simulink model "fuzzy_controller"  (R2015a)
settings: Solver=ode45  StartTime=0.0  StopTime=5  RelTol=1e-3
PreLoadFcn:
  | fuzzy_logic
InitFcn:
  | fuzzy_logic
StartFcn:
  | fuzzy_logic
values from neighbouring files (symbols this model uses):
  A = [zeros(3,3) eye(3); -inv(D_)*G zeros(3,3)]    [double_pend_feedback.m]    (also in fuzzy_logic.m = [zeros(3,3) eye(3); inv(D_)*G zeros(3,3)]; single_pend.m = [0 1 0 0; (g*(M+m))/(l*M) 0 0 b/(l*M); 0 0 0 1; -m*g/M 0 0 -)
  B = [zeros(3,1); inv(D_)*H]    [double_pend_feedback.m]    (also in fuzzy_logic.m; single_pend.m = [0;-1/(l*M); 0 ; 1/M])
  K = double([sol.k1,sol.k2,sol.k3,sol.k4,sol.k5,sol.k6])    [double_pend_feedback.m]    (also in fuzzy_logic.m = lqr2; single_pend.m = [k1 k2 k3 k4])
libraries: fuzblock x1
settings Model: Creator=Nabeel  LastModifiedBy=Nabeel

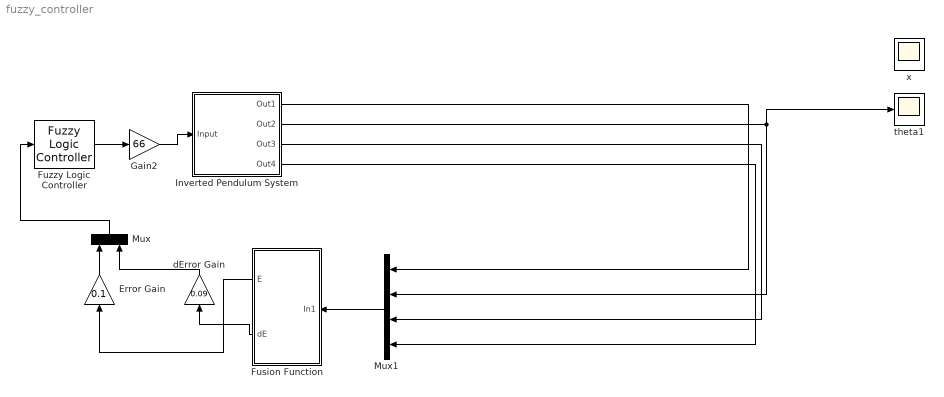
== system fuzzy_controller ==
  Error Gain : Gain  Gain=0.1
  Fusion Function : Subsystem
  Fuzzy Logic Controller : fuzblock/Fuzzy Logic  Controller  fis='MYFUZ.fis'
  Gain2 : Gain  Gain=66
  Inverted Pendulum System : Subsystem
  Mux : Mux  Inputs=2
  Mux1 : Mux
  dError Gain : Gain  Gain=0.09
  theta1 : Scope
      settings: SaveName=theta1
  x : Scope
      settings: SaveName=x
  wires:
  Fuzzy Logic Controller/1 -> Gain2/1
  Gain2/1 -> Inverted Pendulum System/1(Input)
  Fusion Function/1(E) -> Error Gain/1
  Fusion Function/2(dE) -> dError Gain/1
  Mux/1 -> Fuzzy Logic Controller/1
  Error Gain/1 -> Mux/1
  dError Gain/1 -> Mux/2
  Mux1/1 -> Fusion Function/1(In1)
  Inverted Pendulum System/1(Out1) -> Mux1/1
  Inverted Pendulum System/2(Out2) -> Mux1/2, theta1/1
  Inverted Pendulum System/3(Out3) -> Mux1/3
  Inverted Pendulum System/4(Out4) -> Mux1/4

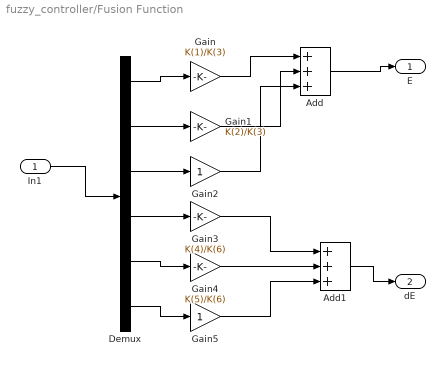
== system fuzzy_controller/Fusion Function ==
  In1 : Inport
  Add : Sum  Inputs=+++
  Add1 : Sum  Inputs=+++
  Demux : Demux  Outputs=6
  Gain : Gain  Gain=K(1)/K(3)
  Gain1 : Gain  Gain=K(2)/K(3)
  Gain2 : Gain
  Gain3 : Gain  Gain=K(4)/K(6)
  Gain4 : Gain  Gain=K(5)/K(6)
  Gain5 : Gain
  E : Outport
  dE : Outport  Port=2
  wires:
  In1/1 -> Demux/1
  Add1/1 -> dE/1
  Add/1 -> E/1
  Demux/6 -> Gain5/1
  Demux/5 -> Gain4/1
  Demux/4 -> Gain3/1
  Demux/3 -> Gain2/1
  Demux/2 -> Gain1/1
  Demux/1 -> Gain/1
  Gain3/1 -> Add1/1
  Gain4/1 -> Add1/2
  Gain5/1 -> Add1/3
  Gain2/1 -> Add/3
  Gain1/1 -> Add/2
  Gain/1 -> Add/1

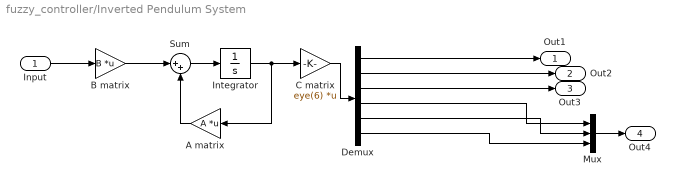
== system fuzzy_controller/Inverted Pendulum System ==
  Input : Inport
  A matrix : Gain  Gain=A  Multiplication=Matrix(K*u)
  B matrix : Gain  Gain=B  Multiplication=Matrix(K*u)
  C matrix : Gain  Gain=eye(6)  Multiplication=Matrix(K*u)
  Demux : Demux  Outputs=6
  Integrator : Integrator  InitialCondition=[0 0.1 0.1 0 0 0]
  Mux : Mux  Inputs=3
  Sum : Sum  Inputs=|++
  Out1 : Outport
  Out2 : Outport  Port=2
  Out3 : Outport  Port=3
  Out4 : Outport  Port=4
  wires:
  Input/1 -> B matrix/1
  A matrix/1 -> Sum/2
  B matrix/1 -> Sum/1
  Sum/1 -> Integrator/1
  Integrator/1 -> C matrix/1, A matrix/1
  C matrix/1 -> Demux/1
  Demux/2 -> Out2/1
  Demux/3 -> Out3/1
  Demux/5 -> Mux/2
  Demux/6 -> Mux/3
  Demux/1 -> Out1/1
  Demux/4 -> Mux/1
  Mux/1 -> Out4/1
